simulink model "StateMachineWithBatchEvents"  (R2021b)
settings: Solver=VariableStepAuto  StartTime=0.0  StopTime=inf  RelTol=1e-3
model workspace (MATLAB code in the model file):
  | % Add the class folders into the path.
  | addpath model
  | addpath utils
  | 
  | %% Loading data from files.
  | % Data for supervisor 1.
  | utils = StateMachineUtils;
  | 
  | % From TCT: Load all events' number.
  | utils = utils.loadEventsInAds('resources/tct/ALLEVENT.ADS');
  | 
  | % From TCT: Disabled events in each state.
  | utils = utils.loadDisabledEventsInPdt('resources/tct/supervisor1/DATA_SIMSUP1_MG1.PDT');
  | 
  | % From TCT: Transition matrix.
  | utils = utils.loadTransitionsInAds('resources/tct/supervisor1/SIMSUP1_MG1.ADS');
  | 
  | % Parameters for the block.
  | encodedStates = StateEncoder.encode(utils.statesArray);
  | 
  | transitions = utils.transitions;
  | 
  | allEvents = utils.eventsArray;
settings Model: Creator=andrerangel  LastModifiedBy=andrerangel

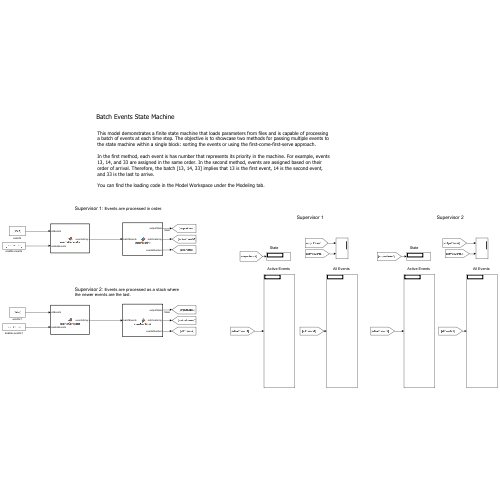
[thumbnail: Simulink's stored preview of the top-level diagram]
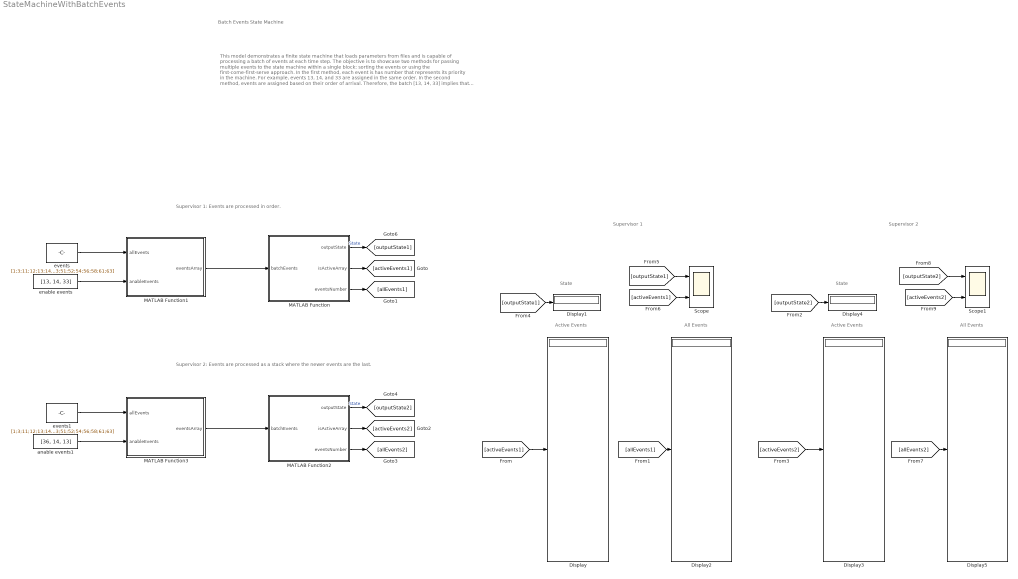
== system StateMachineWithBatchEvents ==
  note: Supervisor 1: Events are processed in order.
  note: Active Events
  note: Supervisor 1
  note: This model demonstrates a finite state machine that loads parameters from files and is capable of processing a batch of events at each time step. The objective is to showcase two methods for passing multiple events to the state machine within a single block: sorting the events or using the first-come-first-serve approach.
      |
      | In the first method, each event is has number that represents its priority in the machine. For example, events 13, 14, and 33 are assigned in the same order. In the second method, events are assigned based on their order of arrival. Therefore, the batch [13, 14, 33] implies that 13 is the first event, 14 is the second event, and 33 is the last to arrive.
      |
      | You can find the loading code in the Model Workspace under the Modeling tab.
  note: State
  note: All Events
  note: Batch Events State Machine
  note: Active Events
  note: Supervisor 2
  note: State
  note: All Events
  note: Supervisor 2: Events are processed as a stack where the newer events are the last.
  Display{,1..5} (6 alike) : Display
  MATLAB Function : MATLAB Function  TreatAsAtomicUnit=on
  MATLAB Function1 : MATLAB Function  TreatAsAtomicUnit=on
  MATLAB Function2 : MATLAB Function  TreatAsAtomicUnit=on
  MATLAB Function3 : MATLAB Function  TreatAsAtomicUnit=on
  Scope : Scope  NumInputPorts=2
  Scope1 : Scope  NumInputPorts=2
  anable events1 : Constant  Value=[36, 14, 13]
  enable events : Constant  Value=[13, 14, 33]
  events : Constant  Value=[1;3;11;12;13;14;16;21;23;25;27;31;32;33;34;36;41;43;51;52;54;56;58;61;63]
  events1 : Constant  Value=[1;3;11;12;13;14;16;21;23;25;27;31;32;33;34;36;41;43;51;52;54;56;58;61;63]
  wires:
  MATLAB Function/1(outputState) -> [outputState1]  "State"
  MATLAB Function/3(eventsNumber) -> [allEvents1]
  [outputState1] -> Scope/1
  [activeEvents1] -> Scope/2
  MATLAB Function/2(isActiveArray) -> [activeEvents1]
  [allEvents1] -> Display2/1
  [activeEvents1] -> Display/1
  [outputState1] -> Display1/1
  events/1 -> MATLAB Function1/1(allEvents)
  enable events/1 -> MATLAB Function1/2(anableEvents)
  MATLAB Function1/1(eventsArray) -> MATLAB Function/1(batchEvents)
  MATLAB Function3/1(eventsArray) -> MATLAB Function2/1(batchEvents)
  anable events1/1 -> MATLAB Function3/2(anableEvents)
  events1/1 -> MATLAB Function3/1(allEvents)
  MATLAB Function2/2(isActiveArray) -> [activeEvents2]
  MATLAB Function2/3(eventsNumber) -> [allEvents2]
  MATLAB Function2/1(outputState) -> [outputState2]  "State"
  [outputState2] -> Display4/1
  [activeEvents2] -> Display3/1
  [allEvents2] -> Display5/1
  [activeEvents2] -> Scope1/2
  [outputState2] -> Scope1/1

== matlab function StateMachineWithBatchEvents/MATLAB Function1 ==
  data: allEvents input; anableEvents input; eventsArray output
function eventsArray = eventsGenerator(allEvents, anableEvents)

[~, indexes] = ismember(anableEvents, allEvents);

eventsArray = zeros(length(allEvents), 1);

eventsArray(indexes) = 1;

== matlab function StateMachineWithBatchEvents/MATLAB Function ==
  data: batchEvents input; outputState output size=[1 1]; isActiveArray output; eventsNumber output; allEvents parameter; transitions parameter; encodedStates parameter
function [outputState, isActiveArray, eventsNumber] = stateMachine( ...
    batchEvents, ...
    allEvents, ...
    transitions, ...
    encodedStates)
% State Machine with parameters from files.
% Receives a batch of events and process one event at time, starting with
% the event of index 1.
% batchEvents: array with 0s and 1s where 1 is the enabled event while 0,
% is disabled event;
% allEvents: numbers of the events;
% transitions: matrix of transitions;
% encodedStates: Encoded states array to be decoded before the pass it to
% StateMachines as an argument.

% Initialize a persistent object. Its value will not be erased as this
% block finishes.
persistent stateMachine

% Assign the persistent object to the StateMachine class with data passed
% as parameters.
if (isempty(stateMachine))
    statesArray = StateEncoder.decode(encodedStates);                        
    stateMachine = StateMachine(statesArray, transitions, allEvents);
end

anabledEvents = allEvents(logical(batchEvents));

% loop through an array of events:
for i=1:length(anabledEvents)
    stateMachine.inputEvent = anabledEvents(i);
end
outputState = stateMachine.currentState.number;
isActiveArray = stateMachine.currentState.activeEvents;
eventsNumber = stateMachine.eventsArray;

== matlab function StateMachineWithBatchEvents/MATLAB Function2 ==
  data: batchEvents input; outputState output size=[1 1]; isActiveArray output; eventsNumber output; allEvents parameter; transitions parameter; encodedStates parameter
function [outputState, isActiveArray, eventsNumber] = stateMachine2( ...
    batchEvents, ...
    allEvents, ...
    transitions, ...
    encodedStates)
% State Machine with parameters from files.
% Receives a batch of events and process one event at time, starting with
% the event of index 1.
% batchEvents: array with 0s and 1s where 1 is the enabled event while 0,
% is disabled event;
% allEvents: numbers of the events;
% transitions: matrix of transitions;
% encodedStates: Encoded states array to be decoded before the pass it to
% StateMachines as an argument.

% Initialize a persistent object. Its value will not be erased as this
% block finishes.
persistent stateMachine
persistent eventsStack

% Assign the persistent object to the StateMachine class with data passed
% as parameters.
if (isempty(stateMachine))
    statesArray = StateEncoder.decode(encodedStates);                        
    stateMachine = StateMachine(statesArray, transitions, allEvents);

    % First run: every event is processed in order.
    eventsStack = allEvents(logical(batchEvents));

    % Loop through an array of events:
    for i=1:length(eventsStack)
        stateMachine.inputEvent = eventsStack(i);
    end

    % Output variables.
    outputState = stateMachine.currentState.number;
    isActiveArray = stateMachine.currentState.activeEvents;
    eventsNumber = stateMachine.eventsArray;
else
    % Get the events' numbers.
    enabledEvents = allEvents(logical(batchEvents));
    
    % Get newer events.
    [logicalPart, indexesPart] = ismember(enabledEvents, eventsStack);
    
    newElements = enabledEvents(indexesPart == 0);

    if ~isempty(newElements)
        % New events stack.
        old = eventsStack(sort(indexesPart(indexesPart ~= 0)));
        eventsStack = [old; newElements];
    end

    % Loop through an array of events:
    for i=1:length(eventsStack)
        stateMachine.inputEvent = eventsStack(i);
    end

    % Output variables.
    outputState = stateMachine.currentState.number;
    isActiveArray = stateMachine.currentState.activeEvents;
    eventsNumber = stateMachine.eventsArray;
end

== matlab function StateMachineWithBatchEvents/MATLAB Function3 ==
  data: allEvents input; anableEvents input; eventsArray output
function eventsArray = eventsGenerator(allEvents, anableEvents)

[~, indexes] = ismember(anableEvents, allEvents);

eventsArray = zeros(length(allEvents), 1);

eventsArray(indexes) = 1;
